simulink model "MCC"  (R2018b)
settings: Solver=FixedStepAuto  StartTime=0.0  StopTime=T_sim  FixedStep=1e-3  RelTol=1e-3
values from neighbouring files (symbols this model uses):
  alfa_echauffement = 4e-3    (= 0.004)    [MCC.m]
  Cn = 104    [MCC.m]
  Cr_ou_pas = input(prompt)    [MCC.m]
  Cref = input(prompt)    [MCC.m]
  Cycle = 0    [MCC.m]
  cycle_vitesse = input(prompt)    [MCC.m]
  delta_teta = 75    [MCC.m]
  Eps_n = 4.69    [MCC.m]
  f = (phi_0*In-Cn)/Omega_n    (= 0.0113704691797)    [MCC.m]
  Imperfection_capteur_ou_pas = input(prompt)    [MCC.m]
  In = 69    [MCC.m]
  J = 0.12    [MCC.m]
  k = f+kc    (= 0.0113704691797)    [MCC.m]
  k1 = 1/cte/(Un/In)    (= 11.6825396825)    [MCC.m]
  k2 = 5*k*to_2/0.3943/phi_0/In*Omega_n    (= 5.00014061884)    [MCC.m]
  kc = 0    [MCC.m]
  Kech = Eps_n/Omega_n/Kgt    (= 0.023058013766)    [MCC.m]
  Kgt = 90/(2*pi/60*1500)    (= 0.572957795131)    [MCC.m]
  L = 6.3e-3    (= 0.0063)    [MCC.m]
  Nn = 3390    [MCC.m]
  Nref = Nn    (= 3390)    [MCC.m]
  Omega_n = Nn*2*pi/60    (= 354.999969856)    [MCC.m]
  phi_0 = (Un-R*In)/Omega_n    (= 1.56574661183)    [MCC.m]
  R = 0.64    [MCC.m]
  R40 = R/(1+alfa_echauffement*delta_teta)    (= 0.492307692308)    [MCC.m]
  rad_V = Eps_n/Omega_n    (= 0.0132112687275)    [MCC.m]
  Rvar_ou_pas = input(prompt)    [MCC.m]
  shunt = 1/240    (= 0.00416666666667)    [MCC.m]
  tau = 1    [MCC.m]
  to_2 = J/k    (= 10.5536542163)    [MCC.m]
  Un = 600    [MCC.m]
  w_0 = 2*pi*30    (= 188.495559215)    [MCC.m]
  xi = sqrt(2)/2    [MCC.m]
libraries: simulink x2
settings Model: Creator=jras  LastModifiedBy=Louis

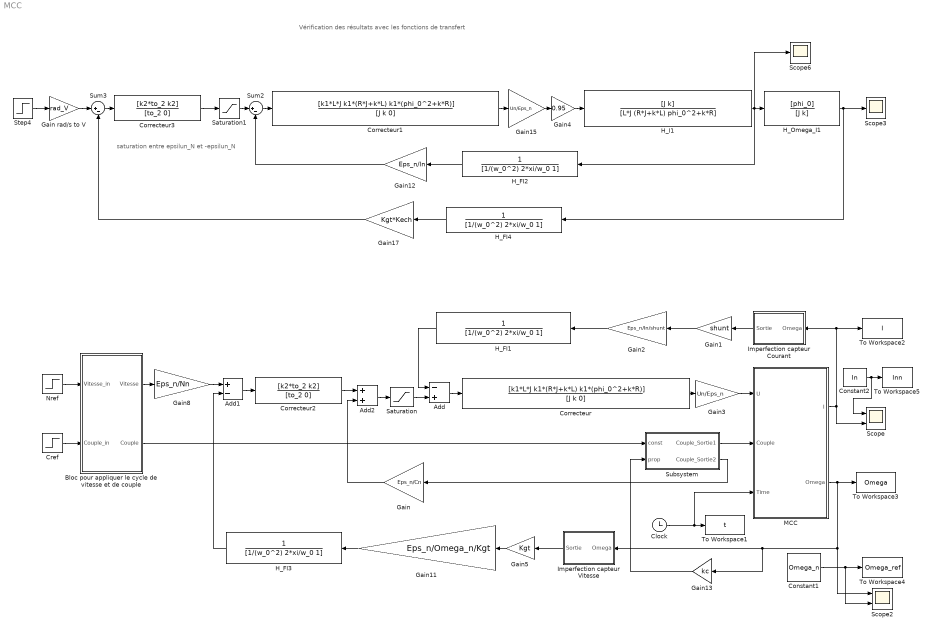
== system MCC ==
  note: Vérification des résultats avec les fonctions de transfert
  note: saturation entre epsilun_N et -epsilun_N
  Add : Sum  Inputs=-+
  Add1 : Sum  Inputs=+-
  Add2 : Sum
  Bloc pour appliquer le cycle de vitesse et de couple : Subsystem
  Clock : Clock
  Constant1 : Constant  Value=Omega_n
  Constant2 : Constant  Value=In
  Correcteur : TransferFcn  Numerator=[k1*L*J k1*(R*J+k*L) k1*(phi_0^2+k*R)]  Denominator=[J k 0]
  Correcteur1 : TransferFcn  Numerator=[k1*L*J k1*(R*J+k*L) k1*(phi_0^2+k*R)]  Denominator=[J k 0]
  Correcteur2 : TransferFcn  Numerator=[k2*to_2 k2]  Denominator=[to_2 0]
  Correcteur3 : TransferFcn  Numerator=[k2*to_2 k2]  Denominator=[to_2 0]
  Cref : Step  Time=5  After=Cref  SampleTime=0
  Gain : Gain  Gain=Eps_n/Cn
  Gain rad/s to V : Gain  Gain=rad_V
  Gain1 : Gain  Gain=shunt
  Gain11 : Gain  Gain=Eps_n/Omega_n/Kgt
  Gain12 : Gain  Gain=Eps_n/In
  Gain13 : Gain  Gain=kc
  Gain15 : Gain  Gain=Un/Eps_n
  Gain17 : Gain  Gain=Kgt*Kech
  Gain2 : Gain  Gain=Eps_n/In/shunt
  Gain3 : Gain  Gain=Un/Eps_n
  Gain4 : Gain  Gain=0.95
  Gain5 : Gain  Gain=Kgt
  Gain8 : Gain  Gain=Eps_n/Nn
  H_FI{1..4} (4 alike) : TransferFcn  Denominator=[1/(w_0^2) 2*xi/w_0 1]
  H_I1 : TransferFcn  Numerator=[J k]  Denominator=[L*J (R*J+k*L) phi_0^2+k*R]
  H_Omega_I1 : TransferFcn  Numerator=[phi_0]  Denominator=[J k]
  Imperfection capteur Courant : Subsystem
  Imperfection capteur Vitesse : Subsystem
  MCC : Subsystem
  Nref : Step  Time=0  After=Nref  SampleTime=0
  Saturation : Saturate  UpperLimit=Eps_n  LowerLimit=-Eps_n
  Saturation1 : Saturate  UpperLimit=Eps_n  LowerLimit=-Eps_n
  Scope : Scope  NumInputPorts=2
  Scope2 : Scope  NumInputPorts=2
  Scope3 : Scope
  Scope6 : Scope
  Step4 : Step  After=Omega_n  SampleTime=0
  Subsystem : Subsystem
  Sum2 : Sum  Inputs=|+-
  Sum3 : Sum  Inputs=|+-
  To Workspace1 : ToWorkspace  VariableName=t  SampleTime=-1
  To Workspace2 : ToWorkspace  VariableName=I  SampleTime=-1
  To Workspace3 : ToWorkspace  VariableName=Omega  SampleTime=-1
  To Workspace4 : ToWorkspace  VariableName=Omega_ref  SampleTime=-1
  To Workspace5 : ToWorkspace  VariableName=Inn  SampleTime=-1
  wires:
  Clock/1 -> To Workspace1/1, MCC/3(Time)
  Saturation/1 -> Add/2
  Gain1/1 -> Gain2/1
  Gain5/1 -> Gain11/1
  MCC/2(Omega) -> Scope2/1, Gain13/1, Imperfection capteur Vitesse/1(Omega), To Workspace3/1
  Gain11/1 -> H_FI3/1
  MCC/1(I) -> Scope/2, To Workspace2/1, Imperfection capteur Courant/1(Omega)
  Constant1/1 -> To Workspace4/1, Scope2/2
  Gain3/1 -> MCC/1(U)
  Gain8/1 -> Add1/1
  Add/1 -> Correcteur/1
  Correcteur/1 -> Gain3/1
  Add2/1 -> Saturation/1
  Correcteur2/1 -> Add2/1
  Add1/1 -> Correcteur2/1
  Constant2/1 -> To Workspace5/1, Scope/1
  Gain2/1 -> H_FI1/1
  H_FI1/1 -> Add/1
  Gain13/1 -> Subsystem/2(prop)
  Subsystem/2(Couple_Sortie2) -> Gain/1
  Subsystem/1(Couple_Sortie1) -> MCC/2(Couple)
  Gain/1 -> Add2/2
  Imperfection capteur Vitesse/1(Sortie) -> Gain5/1
  H_FI3/1 -> Add1/2
  Imperfection capteur Courant/1(Sortie) -> Gain1/1
  Correcteur1/1 -> Gain15/1
  Gain17/1 -> Sum3/2
  Sum2/1 -> Correcteur1/1
  Gain12/1 -> Sum2/2
  Gain4/1 -> H_I1/1
  Correcteur3/1 -> Saturation1/1
  Gain15/1 -> Gain4/1
  Sum3/1 -> Correcteur3/1
  H_FI4/1 -> Gain17/1
  Saturation1/1 -> Sum2/1
  Gain rad/s to V/1 -> Sum3/1
  H_Omega_I1/1 -> Scope3/1, H_FI4/1
  H_FI2/1 -> Gain12/1
  H_I1/1 -> Scope6/1, H_Omega_I1/1, H_FI2/1
  Step4/1 -> Gain rad/s to V/1
  Nref/1 -> Bloc pour appliquer le cycle de vitesse et de couple/1(Vitesse_in)
  Cref/1 -> Bloc pour appliquer le cycle de vitesse et de couple/2(Couple_in)
  Bloc pour appliquer le cycle de vitesse et de couple/1(Vitesse) -> Gain8/1
  Bloc pour appliquer le cycle de vitesse et de couple/2(Couple) -> Subsystem/1(const)

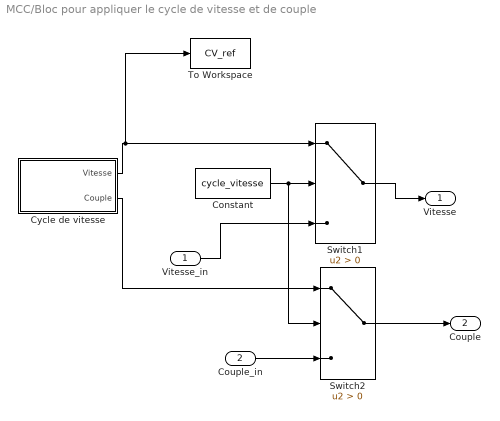
== system MCC/Bloc pour appliquer le cycle de vitesse et de couple ==
  Vitesse_in : Inport
  Couple_in : Inport  Port=2
  Constant : Constant  Value=cycle_vitesse
  "Cycle de vitesse " : Subsystem
  Switch1 : Switch  Criteria=u2 > Threshold
  Switch2 : Switch  Criteria=u2 > Threshold
  To Workspace : ToWorkspace  VariableName=CV_ref  SampleTime=-1
  Vitesse : Outport
  Couple : Outport  Port=2
  wires:
  Couple_in/1 -> Switch2/3
  Constant/1 -> Switch1/2, Switch2/2
  Switch1/1 -> Vitesse/1
  "Cycle de vitesse "/2("Couple ") -> Switch2/1
  "Cycle de vitesse "/1("Vitesse ") -> To Workspace/1, Switch1/1
  Vitesse_in/1 -> Switch1/3
  Switch2/1 -> Couple/1

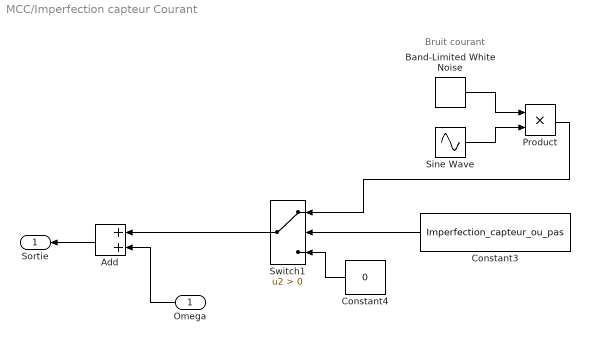
== system MCC/Imperfection capteur Courant ==
  note: Bruit courant
  Omega : Inport
  Add : Sum
  Band-Limited White Noise : simulink/Sources/Band-Limited White Noise  Cov=[0.1]  Ts=0.1  seed=[23341]
  Constant3 : Constant  Value=Imperfection_capteur_ou_pas
  Constant4 : Constant  Value=0
  Product : Product
  Sine Wave : Sin  Amplitude=In/100  Frequency=2*pi*50  SampleTime=0
  Switch1 : Switch  Criteria=u2 > Threshold
  Sortie : Outport
  wires:
  Band-Limited White Noise/1 -> Product/1
  Sine Wave/1 -> Product/2
  Omega/1 -> Add/2
  Add/1 -> Sortie/1
  Product/1 -> Switch1/1
  Switch1/1 -> Add/1
  Constant4/1 -> Switch1/3
  Constant3/1 -> Switch1/2

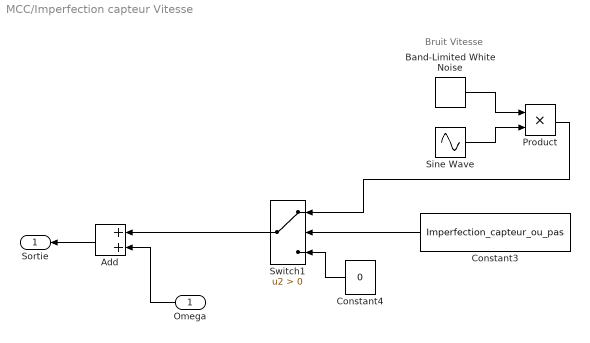
== system MCC/Imperfection capteur Vitesse ==
  note: Bruit Vitesse
  Omega : Inport
  Add : Sum
  Band-Limited White Noise : simulink/Sources/Band-Limited White Noise  Cov=[0.1]  Ts=0.1  seed=[23341]
  Constant3 : Constant  Value=Imperfection_capteur_ou_pas
  Constant4 : Constant  Value=0
  Product : Product
  Sine Wave : Sin  Amplitude=Omega_n/100  Frequency=2*pi*50  SampleTime=0
  Switch1 : Switch  Criteria=u2 > Threshold
  Sortie : Outport
  wires:
  Constant3/1 -> Switch1/2
  Constant4/1 -> Switch1/3
  Switch1/1 -> Add/1
  Product/1 -> Switch1/1
  Add/1 -> Sortie/1
  Omega/1 -> Add/2
  Sine Wave/1 -> Product/2
  Band-Limited White Noise/1 -> Product/1

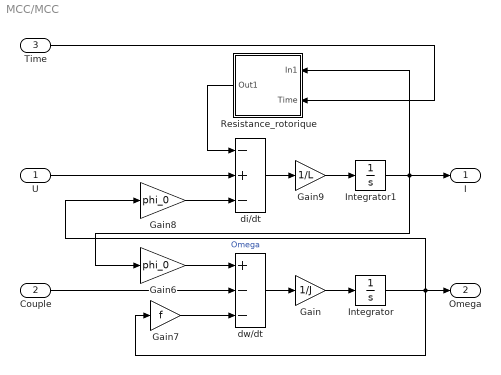
== system MCC/MCC ==
  U : Inport
  Couple : Inport  Port=2
  Time : Inport  Port=3
  Gain : Gain  Gain=1/J
  Gain6 : Gain  Gain=phi_0
  Gain7 : Gain  Gain=f
  Gain8 : Gain  Gain=phi_0
  Gain9 : Gain  Gain=1/L
  Integrator : Integrator
  Integrator1 : Integrator
  Resistance_rotorique : Subsystem
  di/dt : Sum  Inputs=-+-
  dw/dt : Sum  Inputs=+--
  I : Outport
  Omega : Outport  Port=2
  wires:
  Gain9/1 -> Integrator1/1
  Integrator/1 -> Gain8/1, Gain7/1, Omega/1  "Omega"
  Gain6/1 -> dw/dt/1
  Resistance_rotorique/1(Out1) -> di/dt/1
  Integrator1/1 -> I/1, Resistance_rotorique/1(In1), Gain6/1
  di/dt/1 -> Gain9/1
  dw/dt/1 -> Gain/1
  Gain8/1 -> di/dt/3
  Gain7/1 -> dw/dt/3
  Gain/1 -> Integrator/1
  U/1 -> di/dt/2
  Couple/1 -> dw/dt/2
  Time/1 -> Resistance_rotorique/2(Time)

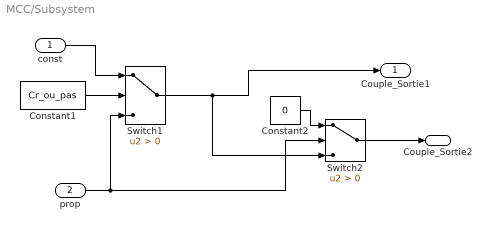
== system MCC/Subsystem ==
  const : Inport
  prop : Inport  Port=2
  Constant1 : Constant  Value=Cr_ou_pas
  Constant2 : Constant  Value=0
  Switch1 : Switch  Criteria=u2 > Threshold
  Switch2 : Switch  Criteria=u2 > Threshold
  Couple_Sortie1 : Outport
  Couple_Sortie2 : Outport  Port=2
  wires:
  prop/1 -> Switch2/2, Switch1/3
  Constant2/1 -> Switch2/1
  Switch1/1 -> Switch2/3, Couple_Sortie1/1
  Switch2/1 -> Couple_Sortie2/1
  Constant1/1 -> Switch1/2
  const/1 -> Switch1/1

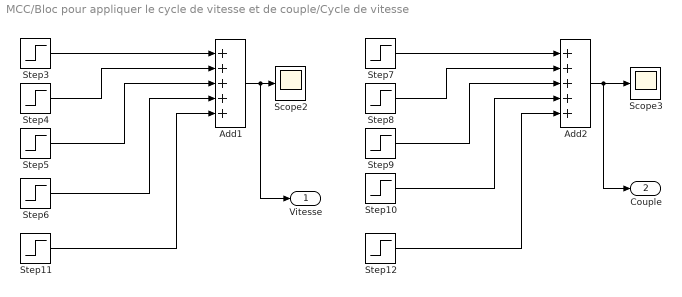
== system MCC/Bloc pour appliquer le cycle de vitesse et de couple/Cycle de vitesse  ==
  Add1 : Sum  Inputs=+++++
  Add2 : Sum  Inputs=+++++
  Scope2 : Scope
  Scope3 : Scope
  Step10 : Step  Time=Cycle+30  After=Cn*(1/100-1/2)  SampleTime=0
  Step11 : Step  Time=Cycle+35  After=-Nn/100  SampleTime=0
  Step12 : Step  Time=Cycle+40  After=-Cn/100  SampleTime=0
  Step3 : Step  Time=Cycle  After=Nn  SampleTime=0
  Step4 : Step  Time=Cycle+10  After=-Nn*2  SampleTime=0
  Step5 : Step  Time=Cycle+20  After=3/2*Nn  SampleTime=0
  Step6 : Step  Time=Cycle+25  After=Nn*(1/100-1/2)  SampleTime=0
  Step7 : Step  Time=Cycle+5  After=Cn  SampleTime=0
  Step8 : Step  Time=Cycle+15  After=-Cn*2  SampleTime=0
  Step9 : Step  Time=Cycle+25  After=3/2*Cn  SampleTime=0
  "Vitesse " : Outport
  "Couple " : Outport  Port=2
  wires:
  Step12/1 -> Add2/5
  Step4/1 -> Add1/2
  Step8/1 -> Add2/2
  Add1/1 -> "Vitesse "/1, Scope2/1
  Step5/1 -> Add1/3
  Step9/1 -> Add2/3
  Step3/1 -> Add1/1
  Step10/1 -> Add2/4
  Step11/1 -> Add1/5
  Add2/1 -> "Couple "/1, Scope3/1
  Step7/1 -> Add2/1
  Step6/1 -> Add1/4

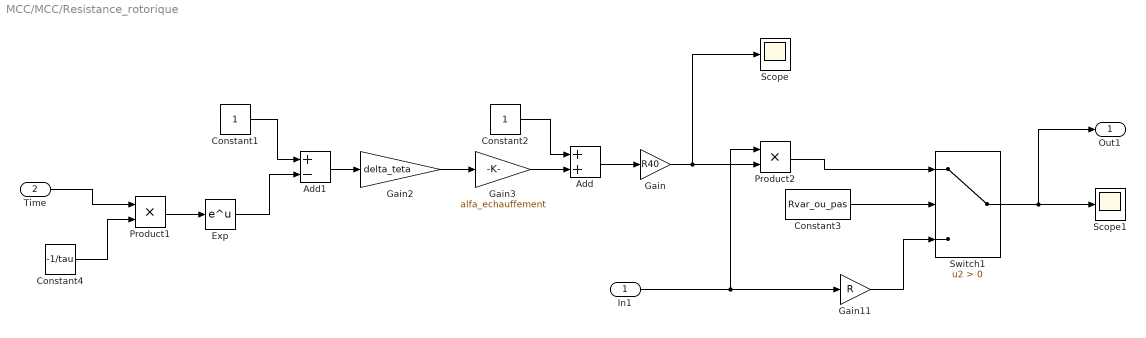
== system MCC/MCC/Resistance_rotorique ==
  In1 : Inport
  Time : Inport  Port=2
  Add : Sum
  Add1 : Sum  Inputs=+-
  Constant1 : Constant
  Constant2 : Constant
  Constant3 : Constant  Value=Rvar_ou_pas
  Constant4 : Constant  Value=-1/tau
  Exp : Math  SaturateOnIntegerOverflow=on
  Gain : Gain  Gain=R40
  Gain11 : Gain  Gain=R
  Gain2 : Gain  Gain=delta_teta
  Gain3 : Gain  Gain=alfa_echauffement
  Product1 : Product
  Product2 : Product
  Scope : Scope
  Scope1 : Scope
  Switch1 : Switch  Criteria=u2 > Threshold
  Out1 : Outport
  wires:
  Gain11/1 -> Switch1/3
  Constant3/1 -> Switch1/2
  Switch1/1 -> Scope1/1, Out1/1
  In1/1 -> Product2/1, Gain11/1
  Time/1 -> Product1/1
  Product1/1 -> Exp/1
  Constant4/1 -> Product1/2
  Exp/1 -> Add1/2
  Constant1/1 -> Add1/1
  Add1/1 -> Gain2/1
  Gain2/1 -> Gain3/1
  Gain3/1 -> Add/2
  Constant2/1 -> Add/1
  Add/1 -> Gain/1
  Gain/1 -> Scope/1, Product2/2
  Product2/1 -> Switch1/1
